simulink model "PMSM_Control"  (R2015b)
settings: Solver=ode1  StartTime=0.0  StopTime=10  FixedStep=0.001  RelTol=1e-3
values from neighbouring files (symbols this model uses):
  c_drag_pro = c_drag*G1.^3*r.^3/G2.^3    [Control_Parameters.m]    (also in M_fil_til_jacob.m; PMSM_State_Space_Parameters.m)
  Den = [2*J_pro*L 2*J_pro*R 3*Kt^2]    [Control_Parameters.m]
  Den1 = [2*J_pro*L 2*Kv*L+2*J_pro*R 3*Kt^2+2*Kv*R]    [Control_Parameters.m]
  G1 = 12    [Control_Parameters.m]    (also in M_fil_til_jacob.m; PMSM_State_Space_Parameters.m)
  G2 = 50    [Control_Parameters.m]    (also in M_fil_til_jacob.m; PMSM_State_Space_Parameters.m)
  J_pro = (m*r^2+J_G2)*(G1/G2)^2 + J_G1    (= 0.281547798877)    [Control_Parameters.m]    (also in M_fil_til_jacob.m; PMSM_State_Space_Parameters.m)
  Ki = (3*alpha^2-((Kp*Kv)/(2*J_pro)-(Kv*R)/(J_pro*L)-(3*Kt^2)/(2*J_pro*L)))*L    (= 0.460640380437)    [Control_Parameters.m]
  Kp = (3*alpha-Kv/J_pro-(R/(2*L)))*L    (= 0.00394985792821)    [Control_Parameters.m]
  Kt = .07329    (= 0.07329)    [Control_Parameters.m]    (also in M_fil_til_jacob.m; PMSM_State_Space_Parameters.m)
  Kv = 0.001    [Control_Parameters.m]    (also in M_fil_til_jacob.m)
  L = 4e-5    (= 4e-05)    [Control_Parameters.m]    (also in M_fil_til_jacob.m; PMSM_State_Space_Parameters.m)
  Num = [3*Kt]    [Control_Parameters.m]
  Num1 = [2*J_pro 2*Kv*L]    [Control_Parameters.m]
  r = 11*.0254/2    (= 0.1397)    [Control_Parameters.m]    (also in M_fil_til_jacob.m; PMSM_State_Space_Parameters.m)
  R = .013/2    (= 0.0065)    [Control_Parameters.m]    (also in M_fil_til_jacob.m; PMSM_State_Space_Parameters.m)
undefined symbols (not defined in the file or in its folder): sigbuilder_block, T_L
libraries: simulink x2
settings Model: Creator=Morten  LastModifiedBy=Morten

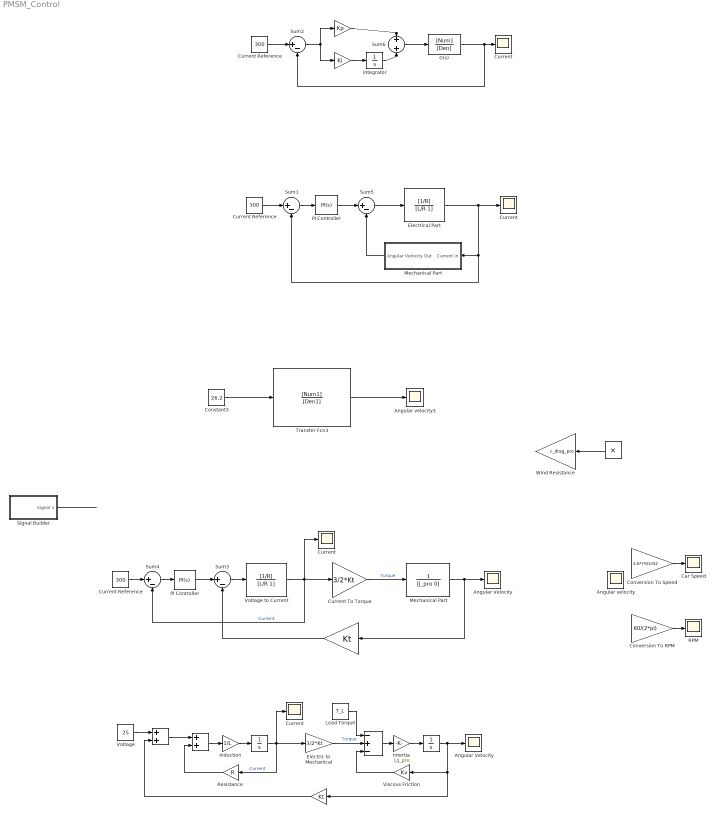
== system PMSM_Control ==
  " " : Product
  "  " : Sum
  "   " : Sum
  "    " : Sum  Inputs=-+-
  " " : Gain  Gain=Ki
  " " : Gain  Gain=Kp
  "             " : Gain  Gain=Kt
  "                          " : Integrator
  "                            " : Gain  Gain=Kt
  "                                     " : Integrator
  "Angular Velocity " : Scope
  "Angular Velocity  " : Scope
  Angular velocity : Scope
  Angular velocity3 : Scope
  Car Speed : Scope
  Constant3 : Constant  Value=26.2
  Conversion To RPM : Gain  Gain=60/(2*pi)
  Conversion To Speed : Gain  Gain=3.6*r*G1/G2
  Current : Scope
  Current Reference : Constant  Value=300
  "Current Reference " : Constant  Value=300
  "Current Reference " : Constant  Value=300
  Current To Torque : Gain  Gain=3/2*Kt
  "Current " : Scope
  "Current " : Scope
  "Current  " : Scope
  Electric to Mechanical : Gain  Gain=3/2*Kt
  Electrical Part : TransferFcn  Numerator=[1/R]  Denominator=[L/R 1]
  G(s) : TransferFcn  Numerator=[Num]  Denominator=[Den]
  Induction : Gain  Gain=1/L
  Integrator : Integrator
  Intertia : Gain  Gain=1/J_pro
  Load Torque : Constant  Value=T_L
  Mechanical Part : TransferFcn  Denominator=[J_pro 0]
  "Mechanical Part " : Subsystem
  PI Controller : simulink/Continuous/PID Controller  Controller=PI  TimeDomain=Continuous-time  SampleTime=-1  IntegratorMethod=Forward Euler  FilterMethod=Forward Euler  Form=Parallel  UseFilter=on  ControllerParametersSource=internal  P=0.00457645136711678  I=2.32438318363822  D=0  N=100  InitialConditionSource=internal  InitialConditionForIntegrator=0  InitialConditionForFilter=0  ExternalReset=none  LimitOutput=off  UpperSaturationLimit=inf  LowerSaturationLimit=-inf  LinearizeAsGain=on  AntiWindupMode=none  Kb=1  TrackingMode=off  Kt=1  PParamMin=[]  PParamMax=[]  IParamMin=[]  IParamMax=[]  DParamMin=[]  DParamMax=[]  NParamMin=[]  NParamMax=[]  KbParamMin=[]  KbParamMax=[]  KtParamMin=[]  KtParamMax=[]  POutMin=[]  POutMax=[]  IOutMin=[]  IOutMax=[]  DOutMin=[]  DOutMax=[]  NOutMin=[]  NOutMax=[]  KbOutMin=[]  KbOutMax=[]  KtOutMin=[]  KtOutMax=[]  IntegratorOutMin=[]  IntegratorOutMax=[]  FilterOutMin=[]  FilterOutMax=[]  SumOutMin=[]  SumOutMax=[]  SumI1OutMin=[]  SumI1OutMax=[]  SumI2OutMin=[]  SumI2OutMax=[]  SumI3OutMin=[]  SumI3OutMax=[]  SumDOutMin=[]  SumDOutMax=[]  SaturationOutMin=[]  SaturationOutMax=[]  IntegratorContinuousStateAttributes=''  IntegratorStateMustResolveToSignalObject=off  IntegratorRTWStateStorageClass=Auto  FilterContinuousStateAttributes=''  FilterStateMustResolveToSignalObject=off  FilterRTWStateStorageClass=Auto  DifferentiatorICPrevScaledInput=0  DifferentiatorOutMin=[]  DifferentiatorOutMax=[]
  "PI Controller " : simulink/Continuous/PID Controller  Controller=PI  TimeDomain=Continuous-time  SampleTime=-1  IntegratorMethod=Forward Euler  FilterMethod=Forward Euler  Form=Parallel  UseFilter=on  ControllerParametersSource=internal  P=0.0039  I=0.4606  D=0  N=100  InitialConditionSource=internal  InitialConditionForIntegrator=0  InitialConditionForFilter=0  ExternalReset=none  LimitOutput=off  UpperSaturationLimit=inf  LowerSaturationLimit=-inf  LinearizeAsGain=on  AntiWindupMode=none  Kb=1  TrackingMode=off  Kt=1  PParamMin=[]  PParamMax=[]  IParamMin=[]  IParamMax=[]  DParamMin=[]  DParamMax=[]  NParamMin=[]  NParamMax=[]  KbParamMin=[]  KbParamMax=[]  KtParamMin=[]  KtParamMax=[]  POutMin=[]  POutMax=[]  IOutMin=[]  IOutMax=[]  DOutMin=[]  DOutMax=[]  NOutMin=[]  NOutMax=[]  KbOutMin=[]  KbOutMax=[]  KtOutMin=[]  KtOutMax=[]  IntegratorOutMin=[]  IntegratorOutMax=[]  FilterOutMin=[]  FilterOutMax=[]  SumOutMin=[]  SumOutMax=[]  SumI1OutMin=[]  SumI1OutMax=[]  SumI2OutMin=[]  SumI2OutMax=[]  SumI3OutMin=[]  SumI3OutMax=[]  SumDOutMin=[]  SumDOutMax=[]  SaturationOutMin=[]  SaturationOutMax=[]  IntegratorContinuousStateAttributes=''  IntegratorStateMustResolveToSignalObject=off  IntegratorRTWStateStorageClass=Auto  FilterContinuousStateAttributes=''  FilterStateMustResolveToSignalObject=off  FilterRTWStateStorageClass=Auto  DifferentiatorICPrevScaledInput=0  DifferentiatorOutMin=[]  DifferentiatorOutMax=[]
  RPM : Scope
  Resistance : Gain  Gain=R
  Signal Builder : Subsystem  Tag=STV Subsys  LoadFcn=sigbuilder_block('load');  StartFcn=sigbuilder_block('start');  StopFcn=sigbuilder_block('stop');  ClipboardFcn=sigbuilder_block('clipboard');  mask(Sigbuilder block){}
      mask help: Simulink:masks:SigbuilderBlock_MD
      mask init:
      | if ~strcmp(get_param(bdroot(gcbh),'SimulationStatus'),'stopped') tuvar = sigbuilder_block('maskInit'); end
      settings: CopyFcn=sigbuilder_block('copy');  DeleteFcn=sigbuilder_block('delete');  ModelCloseFcn=sigbuilder_block('modelClose');  PreSaveFcn=sigbuilder_block('preSave');  PauseFcn=sigbuilder_block('pause');  ContinueFcn=sigbuilder_block('continue');  NameChangeFcn=sigbuilder_block('namechange');  OpenFcn=sigbuilder_block('open',[437.6 199.2 550.4 400 ]);  CloseFcn=sigbuilder_block('close');
      mask Display: plot(0, 0, 100, 100,[2, 2, 32, 32, 2], [68, 8, 8, 68, 68],[32, 2], [38, 38], [32, 19, 2],[53, 60, 44], [32, 17, 17, 2],[16, 16, 31, 31]);txt = getActiveGroup(gcbh);text(2, 100, txt,'verticalAlignment', 'top');
  Sum{1..5} (5 alike) : Sum  Inputs=|+-
  Sum6 : Sum
  Transfer Fcn3 : TransferFcn  Numerator=[Num1]  Denominator=[Den1]
  Viscous Friction : Gain  Gain=Kv
  Voltage : Constant  Value=25
  Voltage to Current : TransferFcn  Numerator=[1/R]  Denominator=[L/R 1]
  Wind Resistance : Gain  Gain=c_drag_pro
  wires:
  "             "/1 -> Sum3/2
  Sum3/1 -> Voltage to Current/1
  Voltage to Current/1 -> Current/1, Current To Torque/1, Sum4/2  "Current"
  Current To Torque/1 -> Mechanical Part/1  "Torque"
  " "/1 -> Wind Resistance/1
  Mechanical Part/1 -> "Angular Velocity "/1, "             "/1
  Conversion To RPM/1 -> RPM/1
  Conversion To Speed/1 -> Car Speed/1
  "PI Controller "/1 -> Sum3/1
  Sum4/1 -> "PI Controller "/1
  PI Controller/1 -> Sum5/1
  Sum1/1 -> PI Controller/1
  Current Reference/1 -> Sum1/1
  "Mechanical Part "/1(Angular Velocity Out) -> Sum5/2
  Sum5/1 -> Electrical Part/1
  Electrical Part/1 -> Sum1/2, "Mechanical Part "/1(Current In), "Current "/1
  Constant3/1 -> Transfer Fcn3/1
  Transfer Fcn3/1 -> Angular velocity3/1
  "Current Reference "/1 -> Sum4/1
  Signal Builder/1(Signal 1) -> ?
  "  "/1 -> "   "/1
  "   "/1 -> Induction/1
  Induction/1 -> "                          "/1
  Resistance/1 -> "   "/2
  "                          "/1 -> Resistance/1, Electric to Mechanical/1, "Current  "/1  "Current"
  Electric to Mechanical/1 -> "    "/2  "Torque"
  Load Torque/1 -> "    "/1
  "    "/1 -> Intertia/1
  Intertia/1 -> "                                     "/1
  Viscous Friction/1 -> "    "/3
  "                                     "/1 -> "Angular Velocity  "/1, "                            "/1, Viscous Friction/1
  "                            "/1 -> "  "/2
  Voltage/1 -> "  "/1
  ? -> Conversion To Speed/1, Conversion To RPM/1, Angular velocity/1
  ? -> " "/1, " "/2
  Sum2/1 -> " "/1, " "/1
  "Current Reference "/1 -> Sum2/1
  G(s)/1 -> Sum2/2, "Current "/1
  " "/1 -> Sum6/1
  " "/1 -> Integrator/1
  Integrator/1 -> Sum6/2
  Sum6/1 -> G(s)/1

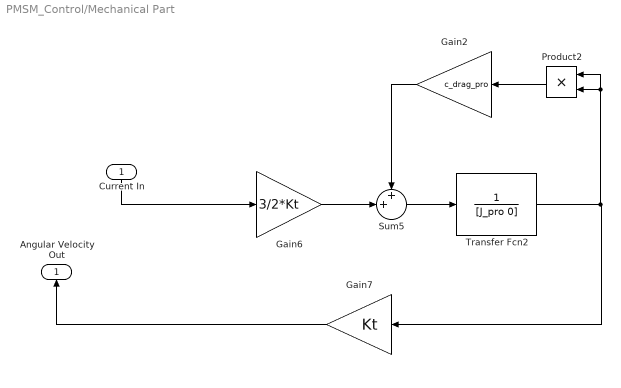
== system PMSM_Control/Mechanical Part  ==
  Current In : Inport
  Gain2 : Gain  Gain=c_drag_pro
  Gain6 : Gain  Gain=3/2*Kt
  Gain7 : Gain  Gain=Kt
  Product2 : Product
  Sum5 : Sum  Inputs=++|
  Transfer Fcn2 : TransferFcn  Denominator=[J_pro 0]
  Angular Velocity Out : Outport
  wires:
  Gain6/1 -> Sum5/2
  Transfer Fcn2/1 -> Product2/2, Product2/1, Gain7/1
  Gain2/1 -> Sum5/1
  Sum5/1 -> Transfer Fcn2/1
  Product2/1 -> Gain2/1
  Gain7/1 -> Angular Velocity Out/1
  Current In/1 -> Gain6/1

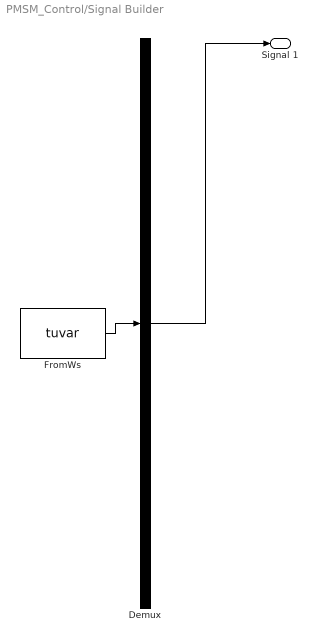
== system PMSM_Control/Signal Builder ==
  Demux : Demux  Tag=STV Demux  Outputs=1
  FromWs : FromWorkspace  Tag=STV FromWs  VariableName=tuvar  SampleTime=0
      SigBuilderData=|
      | common.afterFinalStr = 'Extrapolate'
      | common.sampleTime = 0
      | dataSet.timeRange = [0 10]
      | dataSet.name = 'Group 1'
      | sbobj.Groups.Name = 'Group 1'
      | sbobj.Groups.Signals.Name = 'Signal 1'
      | sbobj.Groups.Signals.XData = [0 0.1 4 6 6 10]
      | sbobj.Groups.Signals.YData = [0 300 300 1 0 0]
  Signal 1 : Outport  Tag=STV Outport
  wires:
  Demux/1 -> Signal 1/1
  FromWs/1 -> Demux/1
